simulink model "heli_q8"  (R2014a)
settings: Solver=ode1  StartTime=0.0  StopTime=inf  FixedStep=0.002  RelTol=1e-3
PostLoadFcn:
  | qc_set_target_type(getConfigSet(bdroot, 'QUARC Default Target Configuration'));
values from neighbouring files (symbols this model uses):
  Joystick_gain_x = 1    [init_heli.m]
  Joystick_gain_y = -1    [init_heli.m]
  K = lqr(A,B,Q,R)    [init_heli.m]
  L_2 = (m_c*l_c-2*m_p*l_h)*g    (= -0.659232)    [init_heli.m]
  L_3 = k_f*l_h    (= 0.0969474)    [init_heli.m]
  P = inv((C_p/(B_p*K_pp-A_p))*B_p)    [init_heli.m]
undefined symbols (not defined in the file or in its folder): HIL, Kpd, Kpp, qc_get_step_size
libraries: simulink_extras x11, quarc_library x4
settings Model: SimulationMode=external  ExtModeTrigDuration=5000  Creator=Rchan  LastModifiedBy=berntjd
settings SolverCC: PositivePriorityOrder=on
settings DataIOCC: SignalLoggingSaveFormat=ModelDataLogs
settings OptimizationCC: ExpressionDepthLimit=2147483647  InitFltsAndDblsToZero=on
settings DebuggingCC: SaveWithParameterizedLinksMsg=none  UnderspecifiedInitializationDetection=Classic  MultiTaskDSMMsg=warning  MultiTaskCondExecSysMsg=none  FcnCallInpInsideContextMsg=UseLocalSettings  StateNameClashWarn=warning
settings RTWCC: SystemTargetFile=quarc_win64.tlc  TemplateMakefile=quarc_default_tmf  Description=QUARC Win64 Target  ProcessScript=quarc_win64_make_rtw_hook
settings STFCustomTargetCC: CPPClassGenCompliant=on
settings GRTTargetCC: ParMdlRefBuildCompliant=off  CompOptLevelCompliant=off  CombineOutputUpdateFcns=off  MatFileLogging=off  GRTInterface=on  ExtMode=on  ExtModeMexFile=quarc_comm

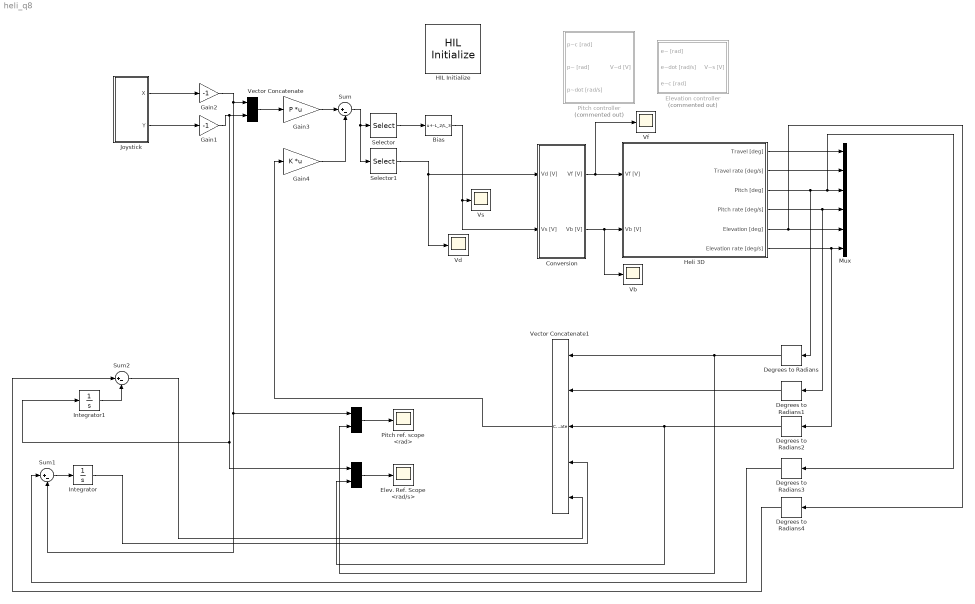
== system heli_q8 ==
  " " : Concatenate
  " " : Concatenate
  Bias : Bias  Bias=-L_2/L_3
  Conversion : Subsystem
  Degrees to Radians{,1..4} (5 alike) : simulink_extras/Transformations/Degrees to Radians
  Elev. Ref. Scope <rad/s> : Scope
      settings: YMin=-0.5  YMax=0.5
  Elevation controller : Subsystem  Commented=on
  Gain1 : Gain  Gain=-1
  Gain2 : Gain  Gain=-1
  Gain3 : Gain  Gain=P  Multiplication=Matrix(K*u) (u vector)
  Gain4 : Gain  Gain=K  Multiplication=Matrix(K*u) (u vector)
  HIL Initialize : quarc_library/Data Acquisition/Generic/Configuration/HIL Initialize  Priority=-99  object_name=HIL-1  board_type=q8_usb  board_number=0  board_options=update_rate=normal;decimation=1  exclusive=off  active=off  hardware_clocks=[0:2]  clock_modes=[]  initial_clock_frequencies=[]  set_clock_params_at_start=off  set_clock_params_at_switch_in=off  set_clock_frequencies_at_start=off  set_clock_frequencies_at_switch_in=off  analog_input_channels=[0:7]  analog_input_maximums=10  analog_input_minimums=-10  set_analog_input_params_at_start=on  set_analog_input_params_at_switch_in=off  analog_output_channels=[0:7]  analog_output_maximums=10  analog_output_minimums=-10  initial_analog_outputs=[0]  final_analog_outputs=[0]  watchdog_analog_outputs=0  set_analog_output_params_at_start=on  set_analog_output_params_at_switch_in=off  set_analog_outputs_at_start=on  set_analog_outputs_at_switch_in=off  set_analog_outputs_at_terminate=on  set_analog_outputs_at_switch_out=off  set_analog_outputs_on_watchdog=off  digital_input_channels=[]  digital_output_channels=[]  digital_output_configuration=[]  initial_digital_outputs=[1]  final_digital_outputs=[1]  watchdog_digital_outputs=[1]  set_digital_output_params_at_start=off  set_digital_output_params_at_switch_in=off  set_digital_outputs_at_start=on  set_digital_outputs_at_switch_in=off  set_digital_outputs_at_terminate=on  set_digital_outputs_at_switch_out=off  set_digital_outputs_on_watchdog=off  encoder_channels=[0:7]  quadrature=[4]  encoder_filter_frequency=[]  initial_encoder_counts=[0]  set_encoder_params_at_start=on  set_encoder_params_at_switch_in=off  set_encoder_counts_at_start=on  set_encoder_counts_at_switch_in=off  pwm_channels=[0:7]  pwm_modes=0  pwm_frequency=99.532799999999995e6/4095  pwm_configuration=[0]  pwm_alignment=[0]  pwm_polarity=[1]  pwm_leading_deadband=[0]  pwm_trailing_deadband=[0]  initial_pwm_outputs=[0]  final_pwm_outputs=[0]  watchdog_pwm_outputs=[0]  set_pwm_params_at_start=on  set_pwm_params_at_switch_in=off  set_pwm_outputs_at_start=on  set_pwm_outputs_at_switch_in=off  set_pwm_outputs_at_terminate=on  set_pwm_outputs_at_switch_out=off  set_pwm_outputs_on_watchdog=off  other_output_channels=[]  initial_other_outputs=[]  final_other_outputs=[]  watchdog_other_outputs=[]  set_other_outputs_at_start=off  set_other_outputs_at_switch_in=off  set_other_outputs_at_terminate=off  set_other_outputs_at_switch_out=off  set_other_outputs_on_watchdog=off
  Heli 3D : Subsystem
  Integrator : Integrator
  Integrator1 : Integrator
  Joystick : Subsystem
  Mux : Mux  Inputs=6
  Pitch controller : Subsystem  Commented=on
  Pitch ref. scope <rad> : Scope
      settings: YMin=-1  YMax=1  SaveName=ScopeData6
  Selector : Selector  InputPortWidth=2  Indices=[1]
  Selector1 : Selector  InputPortWidth=2  Indices=[2]
  Sum : Sum  Inputs=|+-
  Sum1 : Sum  Inputs=|+-
  Sum2 : Sum  Inputs=|+-
  "Vb " : Scope
      settings: YMin=-6  YMax=6  SaveName=ScopeData3
  "Vd " : Scope
      settings: SaveName=ScopeData2
  Vector Concatenate : Concatenate
  Vector Concatenate1 : Concatenate  NumInputs=5
  "Vf " : Scope
      settings: YMin=-6  YMax=6  SaveName=ScopeData4
  Vs : Scope
      settings: YMin=-10  YMax=10
  wires:
  Conversion/2(Vb [V]) -> "Vb "/1, Heli 3D/2(Vb [V])
  Conversion/1(Vf [V]) -> "Vf "/1, Heli 3D/1(Vf [V])
  Heli 3D/1(Travel [deg]) -> Mux/1
  Heli 3D/2(Travel rate [deg/s]) -> Mux/2
  Heli 3D/4(Pitch rate [deg/s]) -> Degrees to Radians1/1, Mux/4
  Heli 3D/6(Elevation rate [deg/s]) -> Degrees to Radians2/1, Mux/6
  Joystick/2(Y) -> Gain1/1
  Joystick/1(X) -> Gain2/1
  Heli 3D/5(Elevation [deg]) -> Degrees to Radians4/1, Mux/5
  Gain1/1 -> " "/1, Integrator1/1, Vector Concatenate/2
  Degrees to Radians2/1 -> " "/2, Vector Concatenate1/3
  Degrees to Radians1/1 -> Vector Concatenate1/2
  Degrees to Radians/1 -> " "/2, Vector Concatenate1/1
  Vector Concatenate/1 -> Gain3/1
  Vector Concatenate1/1 -> Gain4/1
  Gain4/1 -> Sum/2
  Gain3/1 -> Sum/1
  Sum/1 -> Selector1/1, Selector/1
  Selector1/1 -> Conversion/1(Vd [V]), "Vd "/1
  Selector/1 -> Bias/1
  Bias/1 -> Conversion/2(Vs [V]), Vs/1
  " "/1 -> Elev. Ref. Scope <rad/s>/1
  Heli 3D/3(Pitch [deg]) -> Degrees to Radians/1, Degrees to Radians3/1, Mux/3
  Gain2/1 -> Vector Concatenate/1, Sum1/2, " "/1
  " "/1 -> Pitch ref. scope <rad>/1
  Degrees to Radians3/1 -> Sum1/1
  Sum1/1 -> Integrator/1
  Integrator/1 -> Vector Concatenate1/4
  Integrator1/1 -> Sum2/2
  Degrees to Radians4/1 -> Sum2/1
  Sum2/1 -> Vector Concatenate1/5

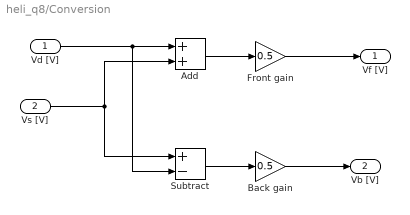
== system heli_q8/Conversion ==
  Vd [V] : Inport
  Vs [V] : Inport  Port=2
  Add : Sum
  Back gain : Gain  Gain=0.5
  Front gain : Gain  Gain=0.5
  Subtract : Sum  Inputs=+-
  Vf [V] : Outport
  Vb [V] : Outport  Port=2
  wires:
  Vd [V]/1 -> Subtract/2, Add/1
  Vs [V]/1 -> Subtract/1, Add/2
  Subtract/1 -> Back gain/1
  Back gain/1 -> Vb [V]/1
  Add/1 -> Front gain/1
  Front gain/1 -> Vf [V]/1

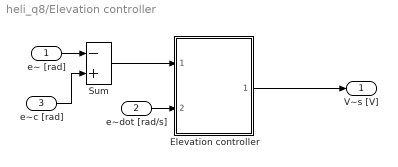
== system heli_q8/Elevation controller ==
  e~ [rad] : Inport
  e~dot [rad/s] : Inport  Port=2
  e~c [rad] : Inport  Port=3
  Elevation controller : Subsystem
  Sum : Sum  Inputs=-+  SaturateOnIntegerOverflow=on  InputSameDT=on  OutDataTypeStr=Inherit: Same as first input
  V~s [V] : Outport  InitialOutput=0
  wires:
  Sum/1 -> Elevation controller/1(e~ [rad])
  Elevation controller/1(V~_s [V]) -> V~s [V]/1
  e~ [rad]/1 -> Sum/1
  e~dot [rad/s]/1 -> Elevation controller/2(e~_dot [rad/s])
  e~c [rad]/1 -> Sum/2

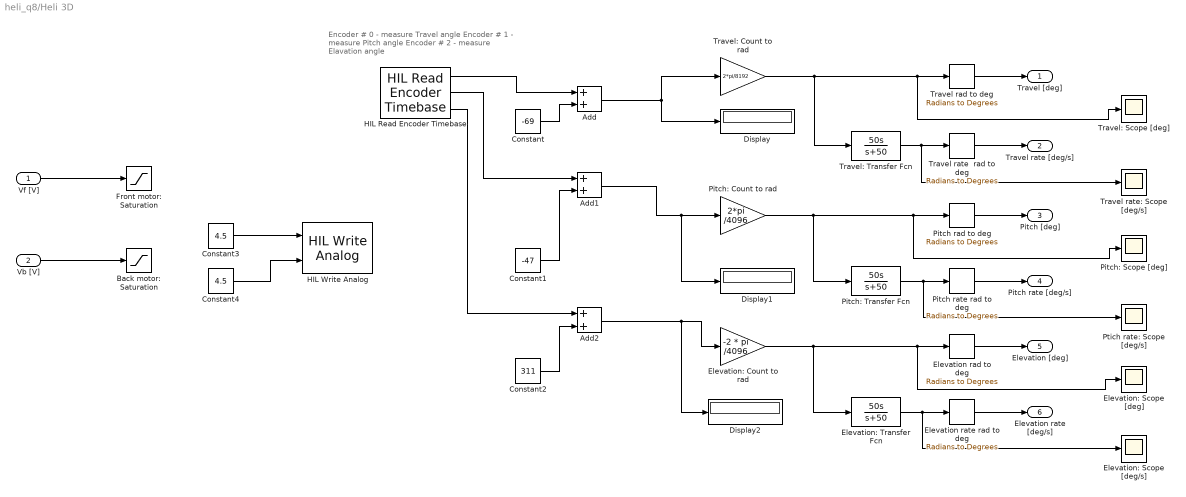
== system heli_q8/Heli 3D ==
  note: Encoder # 0 - measure Travel angle
      | Encoder # 1 - measure Pitch angle
      | Encoder # 2 - measure Elavation angle
  Vf [V] : Inport
  Vb [V] : Inport  Port=2
  Add : Sum
  Add1 : Sum
  Add2 : Sum
  Back motor: Saturation : Saturate  UpperLimit=5  LowerLimit=-5
  Constant : Constant  Value=-69
  Constant1 : Constant  Value=-47
  Constant2 : Constant  Value=311
  Constant3 : Constant  Value=4.5
  Constant4 : Constant  Value=4.5
  Display : Display
      settings: Decimation=2
  Display1 : Display
      settings: Decimation=2
  Display2 : Display
      settings: Decimation=2
  Elevation rad to deg : simulink_extras/Transformations/Radians to Degrees
  Elevation rate rad to deg : simulink_extras/Transformations/Radians to Degrees
  Elevation: Count to rad : Gain  Gain=-2 * pi /4096
  Elevation: Scope [deg/s] : Scope
      settings: YMin=-1  YMax=1  SaveName=ScopeData13
  Elevation: Scope [deg] : Scope
      settings: YMin=-0.5  YMax=0.8  SaveName=ScopeData12
  Elevation: Transfer Fcn : TransferFcn  Numerator=[50 0]  Denominator=[1 50]
  Front motor: Saturation : Saturate  UpperLimit=5  LowerLimit=-5
  HIL Read Encoder Timebase : quarc_library/Data Acquisition/Generic/Timebases/HIL Read Encoder Timebase  object_name=HIL-1  clock=0  channels=[0:2]  samples_in_buffer=max(ceil(1/qc_get_step_size), 1)  active=on  vector_output=off  data_type_mode=Inherit via back propagation  data_type=double
  HIL Write Analog : quarc_library/Data Acquisition/Generic/Immediate I//O/HIL Write Analog  object_name=HIL-1  channels=[0:1]  sample_time=-1  active=off  vector_input=off
  Pitch rad to deg : simulink_extras/Transformations/Radians to Degrees
  Pitch rate rad to deg : simulink_extras/Transformations/Radians to Degrees
  Pitch: Count to rad : Gain  Gain=2*pi /4096
  Pitch: Scope [deg] : Scope
      settings: YMin=-17.5  YMax=2.5  SaveName=ScopeData10
  Pitch: Transfer Fcn : TransferFcn  Numerator=[50 0]  Denominator=[1 50]
  Ptich rate: Scope [deg/s] : Scope
      settings: YMin=-15  YMax=15  SaveName=ScopeData11
  Travel rad to deg : simulink_extras/Transformations/Radians to Degrees
  Travel rate  rad to deg : simulink_extras/Transformations/Radians to Degrees
  Travel rate: Scope [deg/s] : Scope
      settings: YMin=-7.5  YMax=20  SaveName=ScopeData9
  Travel: Count to rad : Gain  Gain=2*pi/8192
  Travel: Scope [deg] : Scope
      settings: YMin=0  YMax=22.5  SaveName=ScopeData8
  Travel: Transfer Fcn : TransferFcn  Numerator=[50 0]  Denominator=[1 50]
  Travel [deg] : Outport
  Travel rate [deg/s] : Outport  Port=2
  Pitch [deg] : Outport  Port=3
  Pitch rate [deg/s] : Outport  Port=4
  Elevation [deg] : Outport  Port=5
  Elevation rate [deg/s] : Outport  Port=6
  wires:
  Travel: Count to rad/1 -> Travel: Transfer Fcn/1, Travel: Scope [deg]/1, Travel rad to deg/1
  Travel: Transfer Fcn/1 -> Travel rate: Scope [deg/s]/1, Travel rate  rad to deg/1
  Pitch: Count to rad/1 -> Pitch: Transfer Fcn/1, Pitch: Scope [deg]/1, Pitch rad to deg/1
  Pitch: Transfer Fcn/1 -> Ptich rate: Scope [deg/s]/1, Pitch rate rad to deg/1
  Elevation: Count to rad/1 -> Elevation: Transfer Fcn/1, Elevation: Scope [deg]/1, Elevation rad to deg/1
  Elevation: Transfer Fcn/1 -> Elevation: Scope [deg/s]/1, Elevation rate rad to deg/1
  Travel rad to deg/1 -> Travel [deg]/1
  Travel rate  rad to deg/1 -> Travel rate [deg/s]/1
  Pitch rad to deg/1 -> Pitch [deg]/1
  Pitch rate rad to deg/1 -> Pitch rate [deg/s]/1
  Elevation rad to deg/1 -> Elevation [deg]/1
  Elevation rate rad to deg/1 -> Elevation rate [deg/s]/1
  Vf [V]/1 -> Front motor: Saturation/1
  Vb [V]/1 -> Back motor: Saturation/1
  HIL Read Encoder Timebase/1 -> Add/1
  Add/1 -> Travel: Count to rad/1, Display/1
  Add1/1 -> Display1/1, Pitch: Count to rad/1
  Add2/1 -> Display2/1, Elevation: Count to rad/1
  HIL Read Encoder Timebase/2 -> Add1/1
  HIL Read Encoder Timebase/3 -> Add2/1
  Constant2/1 -> Add2/2
  Constant1/1 -> Add1/2
  Constant/1 -> Add/2
  Constant3/1 -> HIL Write Analog/1
  Constant4/1 -> HIL Write Analog/2

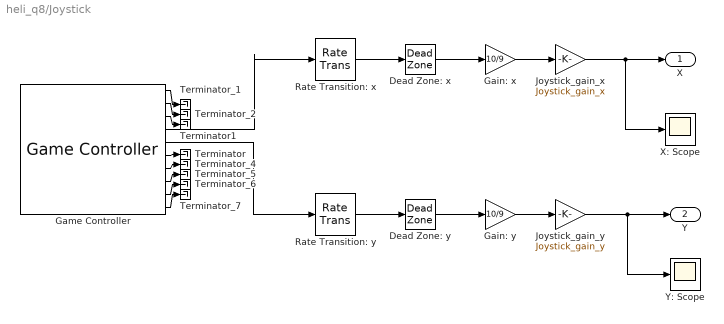
== system heli_q8/Joystick ==
  Dead Zone: x : DeadZone  LowerValue=-0.1  UpperValue=0.1  SaturateOnIntegerOverflow=on
  Dead Zone: y : DeadZone  LowerValue=-0.1  UpperValue=0.1  SaturateOnIntegerOverflow=on
  Gain: x : Gain  Gain=10/9
  Gain: y : Gain  Gain=10/9
  Game Controller : quarc_library/Devices/Peripherals/Target/Game Controller  controller=1  buffer_size=12  deadzone=[]  saturation=[]  sample_time=max(qc_get_step_size, 0.01)  auto_center=off  enabled=on
  Joystick_gain_x : Gain  Gain=Joystick_gain_x
  Joystick_gain_y : Gain  Gain=Joystick_gain_y
  Rate Transition: x : RateTransition
  Rate Transition: y : RateTransition
  Terminator : Terminator
  Terminator1 : Terminator
  Terminator_{1..2,4..7} (6 alike) : Terminator
  X: Scope : Scope
      settings: YMin=-1  YMax=1  SaveName=ScopeData7
  Y: Scope : Scope
      settings: YMin=-10  YMax=10  SaveName=ScopeData5
  X : Outport
  Y : Outport  Port=2
  wires:
  Rate Transition: y/1 -> Dead Zone: y/1
  Rate Transition: x/1 -> Dead Zone: x/1
  Game Controller/5 -> Rate Transition: y/1
  Game Controller/4 -> Rate Transition: x/1
  Game Controller/1 -> Terminator_1/1
  Game Controller/2 -> Terminator_2/1
  Game Controller/7 -> Terminator_4/1
  Game Controller/8 -> Terminator_5/1
  Game Controller/9 -> Terminator_6/1
  Game Controller/10 -> Terminator_7/1
  Game Controller/3 -> Terminator1/1
  Game Controller/6 -> Terminator/1
  Dead Zone: x/1 -> Gain: x/1
  Dead Zone: y/1 -> Gain: y/1
  Gain: x/1 -> Joystick_gain_x/1
  Gain: y/1 -> Joystick_gain_y/1
  Joystick_gain_x/1 -> X/1, X: Scope/1
  Joystick_gain_y/1 -> Y: Scope/1, Y/1

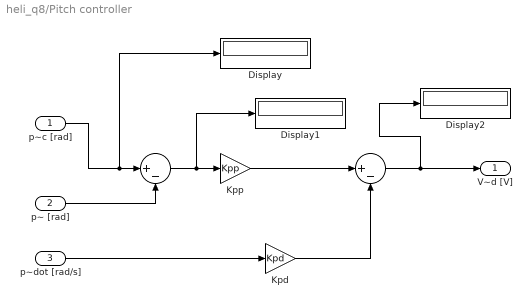
== system heli_q8/Pitch controller ==
  p~c [rad] : Inport
  p~ [rad] : Inport  Port=2
  p~dot [rad/s] : Inport  Port=3
  " " : Sum  Inputs=|+-
  " " : Sum  Inputs=|+-
  Display : Display
      settings: Decimation=5
  Display1 : Display
      settings: Decimation=5
  Display2 : Display
      settings: Decimation=5
  Kpd : Gain  Gain=Kpd
  "Kpp " : Gain  Gain=Kpp
  V~d [V] : Outport  InitialOutput=0
  wires:
  p~c [rad]/1 -> Display/1, " "/1
  p~ [rad]/1 -> " "/2
  " "/1 -> Display1/1, "Kpp "/1
  "Kpp "/1 -> " "/1
  p~dot [rad/s]/1 -> Kpd/1
  " "/1 -> Display2/1, V~d [V]/1
  Kpd/1 -> " "/2

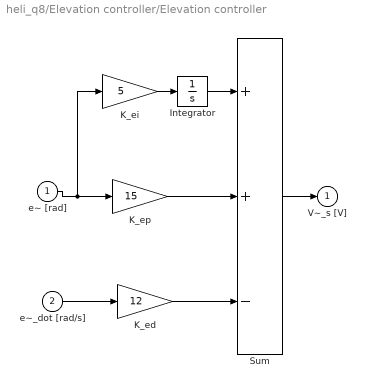
== system heli_q8/Elevation controller/Elevation controller ==
  e~ [rad] : Inport
  e~_dot [rad/s] : Inport  Port=2
  Integrator : Integrator  LimitOutput=on
  K_ed : Gain  Gain=12  SaturateOnIntegerOverflow=on  OutDataTypeStr=Inherit: Same as input  ParamDataTypeStr=Inherit: Same as input
  K_ei : Gain  Gain=5  SaturateOnIntegerOverflow=on  OutDataTypeStr=Inherit: Same as input  ParamDataTypeStr=Inherit: Same as input
  K_ep : Gain  Gain=15  SaturateOnIntegerOverflow=on  OutDataTypeStr=Inherit: Same as input  ParamDataTypeStr=Inherit: Same as input
  Sum : Sum  Inputs=++-  SaturateOnIntegerOverflow=on  InputSameDT=on  OutDataTypeStr=Inherit: Same as first input
  V~_s [V] : Outport  InitialOutput=0
  wires:
  K_ei/1 -> Integrator/1
  Integrator/1 -> Sum/1
  Sum/1 -> V~_s [V]/1
  e~_dot [rad/s]/1 -> K_ed/1
  K_ed/1 -> Sum/3
  K_ep/1 -> Sum/2
  e~ [rad]/1 -> K_ep/1, K_ei/1
